simulink model "watermarking logic"  (R2025a)
settings: Solver=VariableStepAuto  StartTime=0.0  StopTime=50  RelTol=1e-3
settings Model: Creator=Deepak  LastModifiedBy=Deepak

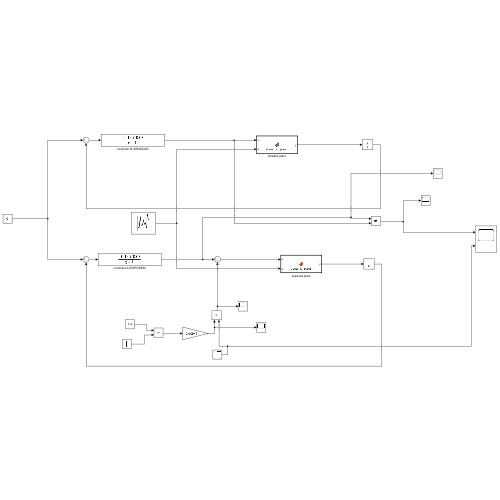
[thumbnail: Simulink's stored preview of the top-level diagram]
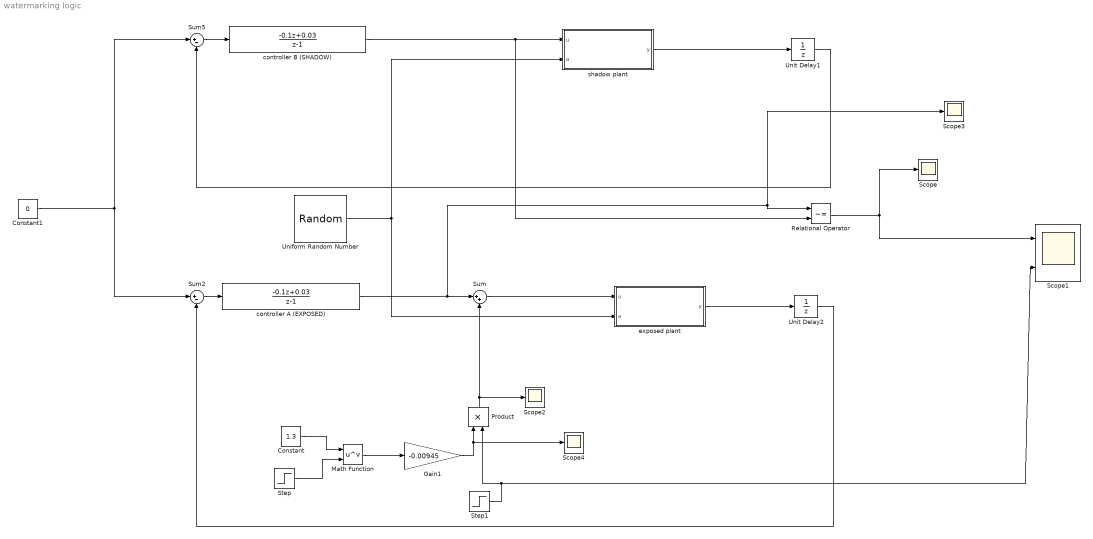
== system watermarking logic ==
  Constant : Constant  Value=1.3
  Constant1 : Constant  Value=0
  Gain1 : Gain  Gain=-0.00945
  Math Function : Math  Operator=pow
  Product : Product
  Relational Operator : RelationalOperator  Operator=~=  OutDataTypeStr=boolean  RndMeth=Simplest  InputSameDT=off
  Scope{,2..4} (4 alike) : Scope
      Scope settings: ActiveDisplayYMinimum=-1  ActiveDisplayYMaximum=1
      Scope2 settings: ActiveDisplayYMinimum=-0.013820625000000001  ActiveDisplayYMaximum=0.0015356249999999997  DataLoggingVariableName=ScopeData2
      Scope3 settings: ActiveDisplayYMinimum=-0.010371933209380926  ActiveDisplayYMaximum=0.067959361601594673  DataLoggingVariableName=ScopeData3
      Scope4 settings: ActiveDisplayYMinimum=-0.0012639375  ActiveDisplayYMaximum=-0.00090956250000000011  DataLoggingVariableName=ScopeData4
  Scope1 : Scope  NumInputPorts=2
      settings: ActiveDisplayYMinimum=-0.12499999999999997  ActiveDisplayYMaximum=1.125
  Step : Step  Time=20  SampleTime=1  VectorParams1D=off  ZeroCross=off
  Step1 : Step  Time=20  SampleTime=1  VectorParams1D=off  ZeroCross=off
  Sum : Sum  Inputs=|++
  Sum2 : Sum  Inputs=|+-
  Sum5 : Sum  Inputs=|+-
  Uniform Random Number : UniformRandomNumber  Minimum=0.01  Maximum=0.1  SampleTime=0.1
  Unit Delay1 : UnitDelay  InitialCondition=1  SampleTime=0.001  HasFrameUpgradeWarning=on
  Unit Delay2 : UnitDelay  InitialCondition=1  SampleTime=0.001  HasFrameUpgradeWarning=on
  controller A (EXPOSED) : DiscreteTransferFcn  Numerator=[-0.1, 0.03]  Denominator=[1, -1]
  controller B (SHADOW) : DiscreteTransferFcn  Numerator=[-0.1, 0.03]  Denominator=[1, -1]
  exposed plant : MATLAB Function  TreatAsAtomicUnit=on
  shadow plant : MATLAB Function  TreatAsAtomicUnit=on
  wires:
  Step1/1 -> Scope1/2, Product/2
  exposed plant/1(y) -> Unit Delay2/1
  Step/1 -> Math Function/2
  controller A (EXPOSED)/1 -> Relational Operator/1, Scope3/1, Sum/1
  Unit Delay1/1 -> Sum5/2
  Constant1/1 -> Sum5/1, Sum2/1
  Sum2/1 -> controller A (EXPOSED)/1
  controller B (SHADOW)/1 -> shadow plant/1(u), Relational Operator/2
  Product/1 -> Sum/2, Scope2/1
  shadow plant/1(y) -> Unit Delay1/1
  Relational Operator/1 -> Scope/1, Scope1/1
  Unit Delay2/1 -> Sum2/2
  Gain1/1 -> Product/1, Scope4/1
  Sum5/1 -> controller B (SHADOW)/1
  Math Function/1 -> Gain1/1
  Constant/1 -> Math Function/1
  Uniform Random Number/1 -> shadow plant/2(a), exposed plant/2(a)
  Sum/1 -> exposed plant/1(u)

== matlab function watermarking logic/shadow plant ==
  data: u input; y output; a input
function y = dynamic_plant(u, a)
    % Discrete-time implementation of G(z) with varying parameter 'a'
    persistent y_1 y_2 u_1 u_2
    
    if isempty(y_1)
        y_1 = 0; y_2 = 0; u_1 = 0; u_2 = 0;
    end
    
    % Difference equation: y(k) = 0.7*y(k-1) - 0.1*y(k-2) + u(k-1) + (a - 1.1)*u(k-2)
    y = 0.7*y_1 - 0.1*y_2 + u_1 + (a - 1.1)*u_2;
    
    y_2 = y_1;
    y_1 = y;
    u_2 = u_1;
    u_1 = u;
end

== matlab function watermarking logic/exposed plant ==
  data: u input; y output; a input
function y = dynamic_plant(u, a)
    % Discrete-time implementation of G(z) with varying parameter 'a'
    persistent y_1 y_2 u_1 u_2
    
    if isempty(y_1)
        y_1 = 0; y_2 = 0; u_1 = 0; u_2 = 0;
    end
    
    % Difference equation: y(k) = 0.7*y(k-1) - 0.1*y(k-2) + u(k-1) + (a - 1.1)*u(k-2)
    y = 0.7*y_1 - 0.1*y_2 + u_1 + (a - 1.1)*u_2;
    
    y_2 = y_1;
    y_1 = y;
    u_2 = u_1;
    u_1 = u;
end
